simulink model "DAQ_v7_IMU_no_Boom_improved_differentiation"  (Simulink 7.8)
settings: Solver=ode3  StartTime=0.0  StopTime=inf  FixedStep=0.001  RelTol=1e-3
InitFcn:
  | DAQParams
model workspace: external: MATLAB File (data not in the file)
undefined symbols (not defined in the file or in its folder): A_dirty_deriv, A_dirty_deriv_IMU, B_dirty_deriv, B_dirty_deriv_IMU, C_dirty_deriv, C_dirty_deriv_IMU, CalParams, D_dirty_deriv, D_dirty_deriv_IMU, Dt_dirty_deriv, Dt_dirty_deriv_IMU, IMU_Alignment_Params, MotorParams, x0_dirty_deriv, x0_dirty_deriv_IMU
libraries: xpcethercatlib x169, dspswit3 x1
(part 1 of 3)
settings Model: xpc_rtwmakecfg_data=_xpcethercatlib_  Creator=hareen  LastModifiedBy=kevinsg  SimulationMode=external  BufferReuse=off
settings DataIOCC: MaxDataPoints=1000000000  SaveFormat=StructureWithTime  SaveState=on
settings OptimizationCC: BlockReduction=off  OptimizeBlockIOStorage=off  BufferReuse=off  ExpressionFolding=off  LocalBlockOutputs=off
settings DebuggingCC: FcnCallInpInsideContextMsg=Use local settings
settings HardwareCC: ProdIntDivRoundTo=Zero  ProdEndianess=LittleEndian  ProdHWDeviceType=Generic->32-bit x86 compatible
settings RTWCC: SystemTargetFile=xpctarget.tlc  TemplateMakefile=xpc_default_tmf  Description=xPC Target  RTWVerbose=off  ProcessScript=xpctarget_make_rtw_hook  RTWCompilerOptimization=On
settings xpcTargetCC: TargetFcnLib=ansi_tfl_table_tmw.mat  TargetFunctionLibrary=XPC_BLAS  CodeExecutionProfiling=off  ParMdlRefBuildCompliant=on  ConcurrentExecutionCompliant=on  CombineSignalStateStructs=off  PortableWordSizes=off  RL32LogBufSizeModifier=10000000  xPCTaskExecutionProfile=off  xPCRL32EventNumber=5000  xPCLoadParamSetFile=off  xPCConcurrentTasks=off  xPCEnableSFAnimation=off

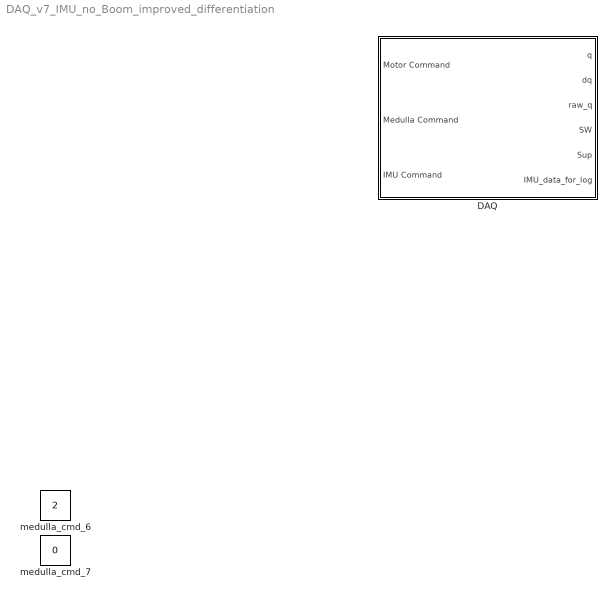
== system DAQ_v7_IMU_no_Boom_improved_differentiation ==
  DAQ : Subsystem
  medulla_cmd_6 : Constant  Value=2
  medulla_cmd_7 : Constant  Value=0

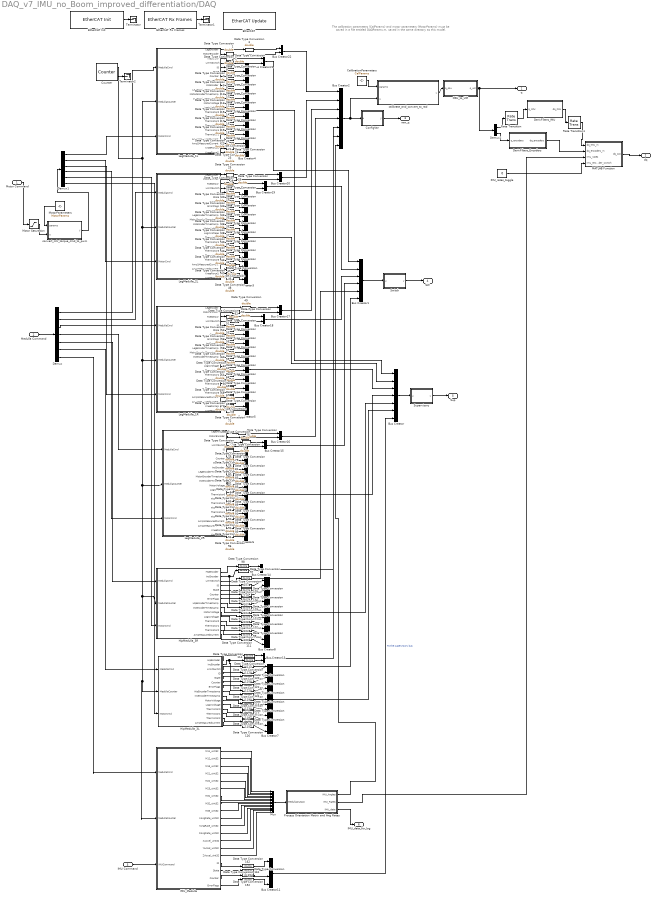
== system DAQ_v7_IMU_no_Boom_improved_differentiation/DAQ ==
  note: The calibration parameters (CalParams) and motor parameters (MotorParams)
      | must be saved in a file entitled DAQParams.m, saved in the same directory
      | as this model.
  Motor Command : Inport
  Medulla Command : Inport  Port=2
  IMU Command : Inport  Port=3
  Bus Creator : BusCreator  Inputs=7
  Bus Creator1 : BusCreator  Inputs=6
  Bus Creator11 : BusCreator
  Bus Creator{13..22} (10 alike) : BusCreator  Inputs=2
  Bus Creator2 : BusCreator  Inputs=7
  Bus Creator{3..6} (4 alike) : BusCreator  Inputs=20
  Bus Creator7 : BusCreator  Inputs=13
  Bus Creator8 : BusCreator  Inputs=13
  CalibrationParameters : Constant  Value=CalParams
  ConfigVar : MATLAB Function  TreatAsAtomicUnit=on
  Counter : dspswit3/Counter  Direction=Up  CountEvent=Free running  CounterSize=User defined  MaxCount=65535  InitialCount=0  Output=Count and Hit  HitValue=32  ResetInput=off  SamplesPerFrame=1  Ts=.001  CntDtype=double  HitDtype=Logical
  Data Type Conversion{1..126,152,154,157..158,161..162} (132 alike) : DataTypeConversion  OutDataTypeStr=double
  Demux : Demux  Outputs=7
  Demux1 : Demux  Outputs=6
  Demux2 : Demux  Outputs=[3 10]
  DerivFilters_Encoders : Subsystem
  DerivFilters_IMU : Subsystem
  EtherCAT : xpcethercatlib/EtherCAT Update   Priority=4  device_id=0  task_id_list=[1]  task_rates=[1]  task_priorities=[1500]  is_async=on  async_rates=20  async_priority=0
  EtherCAT Init : xpcethercatlib/EtherCAT Init   Priority=0  config_file='full_robot_eni_v5_no_boom.xml'  device_id=0  pci_bus=5  pci_slot=5  enaDC=on  errRptLevel=0  sample_time=-1
  EtherCAT Rx Frames : xpcethercatlib/EtherCAT Rx Frames   Priority=1  device_id=0  sample_time=0
  HipMedulla_3L : Subsystem
  HipMedulla_3R : Subsystem
  IMU_Medulla : Subsystem
  IMU_rates_toggle : Constant  Value=0
  LegMedulla_1L : Subsystem
  LegMedulla_1R : Subsystem
  LegMedulla_2L : Subsystem
  LegMedulla_2R : Subsystem
  MATLAB Function : MATLAB Function  TreatAsAtomicUnit=on
  Motor Saturation : Saturate  UpperLimit=50  LowerLimit=-50
  MotorParameters : Constant  Value=MotorParams
  Mux : Mux  Inputs=15
  OSU_to_UM : MATLAB Function  TreatAsAtomicUnit=on
  Process Orientation Matrix and Ang Rates : Subsystem
  Rate Transition : RateTransition  OutPortSampleTimeMultiple=2
  Rate Transition1 : RateTransition  Deterministic=off  OutPortSampleTime=.001
  Supervisory : MATLAB Function  TreatAsAtomicUnit=on
  Switch : MATLAB Function  TreatAsAtomicUnit=on
  Terminator : Terminator
  Terminator1 : Terminator
  Terminator2 : Terminator
  calibrate_and_convert_to_rad : MATLAB Function  TreatAsAtomicUnit=on
  convert_mtr_torque_cmd_to_pwm : MATLAB Function  TreatAsAtomicUnit=on
  q : Outport
  dq : Outport  Port=2
  raw_q : Outport  Port=3
  SW : Outport  Port=4
  Sup : Outport  Port=5
  IMU_data_for_log : Outport  Port=6
  wires:
  LegMedulla_1L/2(MotorEncoder) -> Data Type Conversion1/1
  LegMedulla_1L/3(ToeSensor) -> Data Type Conversion2/1
  LegMedulla_1L/4(LimitSwitch) -> Data Type Conversion4/1
  LegMedulla_1L/5(ID) -> Data Type Conversion5/1
  LegMedulla_1L/6(State) -> Data Type Conversion6/1
  LegMedulla_1L/7(Counter) -> Data Type Conversion7/1
  LegMedulla_1L/8(ErrorFlags) -> Data Type Conversion8/1
  LegMedulla_1L/9(IncEncoder) -> Data Type Conversion9/1
  LegMedulla_1L/10(LegEncoderTimestamp) -> Data Type Conversion10/1
  LegMedulla_1L/11(MotorEncoderTimestamp) -> Data Type Conversion11/1
  LegMedulla_1L/12(IncEncoderTimestamp) -> Data Type Conversion12/1
  LegMedulla_1L/13(MotorVoltage) -> Data Type Conversion13/1
  LegMedulla_1L/14(LogicVoltage) -> Data Type Conversion14/1
  LegMedulla_1L/15(Thermistor0) -> Data Type Conversion15/1
  LegMedulla_1L/16(Thermistor1) -> Data Type Conversion16/1
  LegMedulla_1L/17(Thermistor2) -> Data Type Conversion17/1
  LegMedulla_1L/18(Thermistor3) -> Data Type Conversion18/1
  LegMedulla_1L/19(Thermistor4) -> Data Type Conversion19/1
  LegMedulla_1L/20(Thermistor5) -> Data Type Conversion20/1
  LegMedulla_1L/21(Amp1MeasuredCurrent) -> Data Type Conversion21/1
  LegMedulla_1L/22(Amp2MeasuredCurrent) -> Data Type Conversion22/1
  LegMedulla_1L/23(KneeForce1) -> Data Type Conversion23/1
  LegMedulla_2L/1(LegEncoder) -> Data Type Conversion25/1
  LegMedulla_2L/2(MotorEncoder) -> Data Type Conversion26/1
  LegMedulla_2L/3(ToeSensor) -> Data Type Conversion27/1
  LegMedulla_2L/4(LimitSwitch) -> Data Type Conversion28/1
  LegMedulla_2L/5(ID) -> Data Type Conversion29/1
  LegMedulla_2L/6(State) -> Data Type Conversion30/1
  LegMedulla_2L/7(Counter) -> Data Type Conversion31/1
  LegMedulla_2L/8(ErrorFlags) -> Data Type Conversion32/1
  LegMedulla_2L/9(IncEncoder) -> Data Type Conversion33/1
  LegMedulla_2L/10(LegEncoderTimestamp) -> Data Type Conversion34/1
  LegMedulla_2L/11(MotorEncoderTimestamp) -> Data Type Conversion35/1
  LegMedulla_2L/12(IncEncoderTimestamp) -> Data Type Conversion36/1
  LegMedulla_2L/13(MotorVoltage) -> Data Type Conversion37/1
  LegMedulla_2L/14(LogicVoltage) -> Data Type Conversion38/1
  LegMedulla_2L/15(Thermistor0) -> Data Type Conversion39/1
  LegMedulla_2L/16(Thermistor1) -> Data Type Conversion40/1
  LegMedulla_2L/17(Thermistor2) -> Data Type Conversion41/1
  LegMedulla_2L/18(Thermistor3) -> Data Type Conversion42/1
  LegMedulla_2L/19(Thermistor4) -> Data Type Conversion43/1
  LegMedulla_2L/20(Thermistor5) -> Data Type Conversion44/1
  LegMedulla_2L/21(Amp1MeasuredCurrent) -> Data Type Conversion45/1
  LegMedulla_2L/22(Amp2MeasuredCurrent) -> Data Type Conversion46/1
  LegMedulla_2L/23(KneeForce1) -> Data Type Conversion47/1
  LegMedulla_1L/24(KneeForce2) -> Data Type Conversion24/1
  LegMedulla_2L/24(KneeForce2) -> Data Type Conversion48/1
  LegMedulla_1R/3(ToeSensor) -> Data Type Conversion51/1
  LegMedulla_1R/4(LimitSwitch) -> Data Type Conversion52/1
  LegMedulla_1R/5(ID) -> Data Type Conversion53/1
  LegMedulla_1R/6(State) -> Data Type Conversion54/1
  LegMedulla_1R/7(Counter) -> Data Type Conversion55/1
  LegMedulla_1R/8(ErrorFlags) -> Data Type Conversion56/1
  LegMedulla_1R/9(IncEncoder) -> Data Type Conversion57/1
  LegMedulla_1R/10(LegEncoderTimestamp) -> Data Type Conversion58/1
  LegMedulla_1R/11(MotorEncoderTimestamp) -> Data Type Conversion59/1
  LegMedulla_1R/12(IncEncoderTimestamp) -> Data Type Conversion60/1
  LegMedulla_1R/13(MotorVoltage) -> Data Type Conversion61/1
  LegMedulla_1R/14(LogicVoltage) -> Data Type Conversion62/1
  LegMedulla_1R/15(Thermistor0) -> Data Type Conversion63/1
  LegMedulla_1R/16(Thermistor1) -> Data Type Conversion64/1
  LegMedulla_1R/17(Thermistor2) -> Data Type Conversion65/1
  LegMedulla_1R/18(Thermistor3) -> Data Type Conversion66/1
  LegMedulla_1R/19(Thermistor4) -> Data Type Conversion67/1
  LegMedulla_1R/20(Thermistor5) -> Data Type Conversion68/1
  LegMedulla_1R/21(Amp1MeasuredCurrent) -> Data Type Conversion69/1
  LegMedulla_1R/22(Amp2MeasuredCurrent) -> Data Type Conversion70/1
  LegMedulla_1R/23(KneeForce1) -> Data Type Conversion71/1
  LegMedulla_2R/4(LimitSwitch) -> Data Type Conversion76/1
  LegMedulla_2R/5(ID) -> Data Type Conversion77/1
  LegMedulla_2R/6(State) -> Data Type Conversion78/1
  LegMedulla_2R/7(Counter) -> Data Type Conversion79/1
  LegMedulla_2R/8(ErrorFlags) -> Data Type Conversion80/1
  LegMedulla_2R/9(IncEncoder) -> Data Type Conversion81/1
  LegMedulla_2R/10(LegEncoderTimestamp) -> Data Type Conversion82/1
  LegMedulla_2R/11(MotorEncoderTimestamp) -> Data Type Conversion83/1
  LegMedulla_2R/12(IncEncoderTimestamp) -> Data Type Conversion84/1
  LegMedulla_2R/13(MotorVoltage) -> Data Type Conversion85/1
  LegMedulla_2R/14(LogicVoltage) -> Data Type Conversion86/1
  LegMedulla_2R/15(Thermistor0) -> Data Type Conversion87/1
  LegMedulla_2R/16(Thermistor1) -> Data Type Conversion88/1
  LegMedulla_2R/17(Thermistor2) -> Data Type Conversion89/1
  LegMedulla_2R/18(Thermistor3) -> Data Type Conversion90/1
  LegMedulla_2R/19(Thermistor4) -> Data Type Conversion91/1
  LegMedulla_2R/20(Thermistor5) -> Data Type Conversion92/1
  LegMedulla_2R/21(Amp1MeasuredCurrent) -> Data Type Conversion93/1
  LegMedulla_2R/22(Amp2MeasuredCurrent) -> Data Type Conversion94/1
  LegMedulla_2R/23(KneeForce1) -> Data Type Conversion95/1
  LegMedulla_1R/24(KneeForce2) -> Data Type Conversion72/1
  LegMedulla_2R/24(KneeForce2) -> Data Type Conversion96/1
  Counter/1 -> LegMedulla_1L/2(MedullaCounter), LegMedulla_2L/2(MedullaCounter), LegMedulla_1R/2(MedullaCounter), LegMedulla_2R/2(MedullaCounter), HipMedulla_3R/2(MedullaCounter), HipMedulla_3L/2(MedullaCounter), IMU_Medulla/2(MedullaCounter)
  Medulla Command/1 -> Demux/1
  Demux/1 -> LegMedulla_1L/1(MedullaCmd)
  Demux/2 -> LegMedulla_2L/1(MedullaCmd)
  Demux/3 -> LegMedulla_1R/1(MedullaCmd)
  Demux/4 -> LegMedulla_2R/1(MedullaCmd)
  Demux/5 -> HipMedulla_3R/1(MedullaCmd)
  Demux/6 -> HipMedulla_3L/1(MedullaCmd)
  Demux/7 -> IMU_Medulla/1(MedullaCmd)
  Demux1/1 -> LegMedulla_1L/3(MotorCmd)
  Demux1/2 -> LegMedulla_2L/3(MotorCmd)
  Demux1/3 -> LegMedulla_1R/3(MotorCmd)
  Demux1/4 -> LegMedulla_2R/3(MotorCmd)
  Demux1/5 -> HipMedulla_3R/3(MotorCmd)
  Demux1/6 -> HipMedulla_3L/3(MotorCmd)
  EtherCAT Init/1 -> Terminator/1
  EtherCAT Rx Frames/1 -> Terminator1/1
  Counter/2 -> Terminator2/1
  LegMedulla_2R/1(LegEncoder) -> Data Type Conversion73/1
  LegMedulla_2R/2(MotorEncoder) -> Data Type Conversion74/1
  LegMedulla_2R/3(ToeSensor) -> Data Type Conversion75/1
  Data Type Conversion51/1 -> Bus Creator18/1
  Data Type Conversion52/1 -> Bus Creator18/2
  Data Type Conversion53/1 -> Bus Creator5/1
  Data Type Conversion54/1 -> Bus Creator5/2
  Data Type Conversion55/1 -> Bus Creator5/3
  Data Type Conversion56/1 -> Bus Creator5/4
  Data Type Conversion57/1 -> Bus Creator5/5
  Data Type Conversion58/1 -> Bus Creator5/6
  Data Type Conversion59/1 -> Bus Creator5/7
  Data Type Conversion60/1 -> Bus Creator5/8
  Data Type Conversion61/1 -> Bus Creator5/9
  Data Type Conversion62/1 -> Bus Creator5/10
  Data Type Conversion63/1 -> Bus Creator5/11
  Data Type Conversion64/1 -> Bus Creator5/12
  Data Type Conversion65/1 -> Bus Creator5/13
  Data Type Conversion66/1 -> Bus Creator5/14
  Data Type Conversion67/1 -> Bus Creator5/15
  Data Type Conversion68/1 -> Bus Creator5/16
  Data Type Conversion69/1 -> Bus Creator5/17
  Data Type Conversion70/1 -> Bus Creator5/18
  Data Type Conversion71/1 -> Bus Creator5/19
  Data Type Conversion72/1 -> Bus Creator5/20
  Data Type Conversion73/1 -> Bus Creator16/1
  Data Type Conversion74/1 -> Bus Creator16/2
  Data Type Conversion75/1 -> Bus Creator15/1
  Data Type Conversion76/1 -> Bus Creator15/2
  Data Type Conversion77/1 -> Bus Creator6/1
  Data Type Conversion78/1 -> Bus Creator6/2
  Data Type Conversion79/1 -> Bus Creator6/3
  Data Type Conversion80/1 -> Bus Creator6/4
  Data Type Conversion81/1 -> Bus Creator6/5
  Data Type Conversion82/1 -> Bus Creator6/6
  Data Type Conversion83/1 -> Bus Creator6/7
  Data Type Conversion84/1 -> Bus Creator6/8
  Data Type Conversion85/1 -> Bus Creator6/9
  Data Type Conversion86/1 -> Bus Creator6/10
  Data Type Conversion87/1 -> Bus Creator6/11
  Data Type Conversion88/1 -> Bus Creator6/12
  Data Type Conversion89/1 -> Bus Creator6/13
  Data Type Conversion90/1 -> Bus Creator6/14
  Data Type Conversion91/1 -> Bus Creator6/15
  Data Type Conversion92/1 -> Bus Creator6/16
  Data Type Conversion93/1 -> Bus Creator6/17
  Data Type Conversion94/1 -> Bus Creator6/18
  Data Type Conversion95/1 -> Bus Creator6/19
  Data Type Conversion96/1 -> Bus Creator6/20
  Data Type Conversion111/1 -> Bus Creator8/13
  Motor Command/1 -> Motor Saturation/1
  MotorParameters/1 -> convert_mtr_torque_cmd_to_pwm/1(params)
  Motor Saturation/1 -> convert_mtr_torque_cmd_to_pwm/2(u)
  LegMedulla_1R/2(MotorEncoder) -> Data Type Conversion50/1
  LegMedulla_1L/1(LegEncoder) -> Data Type Conversion3/1
  LegMedulla_1R/1(LegEncoder) -> Data Type Conversion49/1
  Bus Creator22/1 -> Bus Creator2/1
  Bus Creator20/1 -> Bus Creator2/2
  Bus Creator17/1 -> Bus Creator2/3
  Bus Creator16/1 -> Bus Creator2/4
  Bus Creator14/1 -> Bus Creator2/5
  Bus Creator18/1 -> Bus Creator1/3
  Bus Creator19/1 -> Bus Creator1/2
  Bus Creator21/1 -> Bus Creator1/1
  Bus Creator15/1 -> Bus Creator1/4
  Data Type Conversion3/1 -> Bus Creator22/1
  Data Type Conversion1/1 -> Bus Creator22/2
  Data Type Conversion2/1 -> Bus Creator21/1
  Data Type Conversion4/1 -> Bus Creator21/2
  Data Type Conversion5/1 -> Bus Creator4/1
  Data Type Conversion6/1 -> Bus Creator4/2
  Data Type Conversion7/1 -> Bus Creator4/3
  Data Type Conversion8/1 -> Bus Creator4/4
  Data Type Conversion9/1 -> Bus Creator4/5
  Data Type Conversion10/1 -> Bus Creator4/6
  Data Type Conversion11/1 -> Bus Creator4/7
  Data Type Conversion12/1 -> Bus Creator4/8
  Data Type Conversion13/1 -> Bus Creator4/9
  Data Type Conversion14/1 -> Bus Creator4/10
  Data Type Conversion15/1 -> Bus Creator4/11
  Data Type Conversion16/1 -> Bus Creator4/12
  Data Type Conversion17/1 -> Bus Creator4/13
  Data Type Conversion18/1 -> Bus Creator4/14
  Data Type Conversion19/1 -> Bus Creator4/15
  Data Type Conversion20/1 -> Bus Creator4/16
  Data Type Conversion21/1 -> Bus Creator4/17
  Data Type Conversion22/1 -> Bus Creator4/18
  Data Type Conversion23/1 -> Bus Creator4/19
  Data Type Conversion24/1 -> Bus Creator4/20
  Data Type Conversion25/1 -> Bus Creator20/1
  Data Type Conversion26/1 -> Bus Creator20/2
  Data Type Conversion27/1 -> Bus Creator19/1
  Data Type Conversion28/1 -> Bus Creator19/2
  Data Type Conversion29/1 -> Bus Creator3/1
  Data Type Conversion30/1 -> Bus Creator3/2
  Data Type Conversion31/1 -> Bus Creator3/3
  Data Type Conversion32/1 -> Bus Creator3/4
  Data Type Conversion33/1 -> Bus Creator3/5
  Data Type Conversion34/1 -> Bus Creator3/6
  Data Type Conversion35/1 -> Bus Creator3/7
  Data Type Conversion36/1 -> Bus Creator3/8
  Data Type Conversion37/1 -> Bus Creator3/9
  Data Type Conversion38/1 -> Bus Creator3/10
  Data Type Conversion39/1 -> Bus Creator3/11
  Data Type Conversion40/1 -> Bus Creator3/12
  Data Type Conversion41/1 -> Bus Creator3/13
  Data Type Conversion42/1 -> Bus Creator3/14
  Data Type Conversion43/1 -> Bus Creator3/15
  Data Type Conversion44/1 -> Bus Creator3/16
  Data Type Conversion45/1 -> Bus Creator3/17
  Data Type Conversion46/1 -> Bus Creator3/18
  Data Type Conversion47/1 -> Bus Creator3/19
  Data Type Conversion48/1 -> Bus Creator3/20
  Data Type Conversion49/1 -> Bus Creator17/1
  Data Type Conversion50/1 -> Bus Creator17/2
  convert_mtr_torque_cmd_to_pwm/1(y) -> Demux1/1
  Data Type Conversion99/1 -> Bus Creator8/12
  Data Type Conversion100/1 -> Bus Creator8/11
  Data Type Conversion102/1 -> Bus Creator8/10
  Data Type Conversion103/1 -> Bus Creator8/9
  Data Type Conversion101/1 -> Bus Creator8/8
  Data Type Conversion108/1 -> Bus Creator8/7
  Data Type Conversion109/1 -> Bus Creator8/6
  Data Type Conversion104/1 -> Bus Creator8/5
  Data Type Conversion106/1 -> Bus Creator8/4
  Data Type Conversion107/1 -> Bus Creator8/3
  Data Type Conversion105/1 -> Bus Creator8/2
  Data Type Conversion110/1 -> Bus Creator8/1
  Data Type Conversion97/1 -> Bus Creator14/2
  Data Type Conversion98/1 -> Bus Creator14/1
  HipMedulla_3R/1(HipEncoder) -> Data Type Conversion98/1
  HipMedulla_3R/2(IncEncoder) -> Data Type Conversion97/1, Data Type Conversion104/1
  Data Type Conversion157/1 -> Bus Creator1/5
  HipMedulla_3R/3(LimitSwitch) -> Data Type Conversion157/1
  HipMedulla_3R/4(ID) -> Data Type Conversion110/1
  HipMedulla_3R/5(State) -> Data Type Conversion105/1
  HipMedulla_3R/6(Counter) -> Data Type Conversion107/1
  HipMedulla_3R/7(ErrorFlags) -> Data Type Conversion106/1
  HipMedulla_3R/8(HipEncoderTimestamp) -> Data Type Conversion109/1
  HipMedulla_3R/9(IncEncoderTimestamp) -> Data Type Conversion108/1
  HipMedulla_3R/10(MotorVoltage) -> Data Type Conversion101/1
  HipMedulla_3R/11(LogicVoltage) -> Data Type Conversion103/1
  HipMedulla_3R/12(Thermistor0) -> Data Type Conversion102/1
  HipMedulla_3R/13(Thermistor1) -> Data Type Conversion100/1
  HipMedulla_3R/14(Thermistor2) -> Data Type Conversion99/1
  HipMedulla_3R/15(AmpMeasuredCurrent) -> Data Type Conversion111/1
  Bus Creator13/1 -> Bus Creator2/6
  HipMedulla_3L/3(LimitSwitch) -> Data Type Conversion112/1
  Data Type Conversion112/1 -> Bus Creator1/6
  Data Type Conversion113/1 -> Bus Creator13/2
  Data Type Conversion114/1 -> Bus Creator13/1
  HipMedulla_3L/1(HipEncoder) -> Data Type Conversion114/1
  HipMedulla_3L/2(IncEncoder) -> Data Type Conversion113/1, Data Type Conversion119/1
  Data Type Conversion126/1 -> Bus Creator7/13
  Data Type Conversion158/1 -> Bus Creator7/12
  Data Type Conversion115/1 -> Bus Creator7/11
  Data Type Conversion117/1 -> Bus Creator7/10
  Data Type Conversion118/1 -> Bus Creator7/9
  Data Type Conversion116/1 -> Bus Creator7/8
  Data Type Conversion123/1 -> Bus Creator7/7
  Data Type Conversion124/1 -> Bus Creator7/6
  Data Type Conversion119/1 -> Bus Creator7/5
  Data Type Conversion121/1 -> Bus Creator7/4
  Data Type Conversion122/1 -> Bus Creator7/3
  Data Type Conversion120/1 -> Bus Creator7/2
  Data Type Conversion125/1 -> Bus Creator7/1
  HipMedulla_3L/4(ID) -> Data Type Conversion125/1
  HipMedulla_3L/5(State) -> Data Type Conversion120/1
  HipMedulla_3L/6(Counter) -> Data Type Conversion122/1
  HipMedulla_3L/7(ErrorFlags) -> Data Type Conversion121/1
  HipMedulla_3L/8(HipEncoderTimestamp) -> Data Type Conversion124/1
  HipMedulla_3L/9(IncEncoderTimestamp) -> Data Type Conversion123/1
  HipMedulla_3L/10(MotorVoltage) -> Data Type Conversion116/1
  HipMedulla_3L/11(LogicVoltage) -> Data Type Conversion118/1
  HipMedulla_3L/12(Thermistor0) -> Data Type Conversion117/1
  HipMedulla_3L/13(Thermistor1) -> Data Type Conversion115/1
  HipMedulla_3L/14(Thermistor2) -> Data Type Conversion158/1
  HipMedulla_3L/15(AmpMeasuredCurrent) -> Data Type Conversion126/1
  Bus Creator8/1 -> Bus Creator/5
  Bus Creator6/1 -> Bus Creator/4
  Bus Creator5/1 -> Bus Creator/3
  Bus Creator3/1 -> Bus Creator/2
  Bus Creator4/1 -> Bus Creator/1
  Bus Creator7/1 -> Bus Creator/6
  Bus Creator1/1 -> Switch/1(u)
  Bus Creator/1 -> Supervisory/1(u)
  Switch/1(y) -> SW/1
  Supervisory/1(y) -> Sup/1
  Bus Creator2/1 -> ConfigVar/1(u), calibrate_and_convert_to_rad/2(u)
  ConfigVar/1(y) -> raw_q/1
  CalibrationParameters/1 -> calibrate_and_convert_to_rad/1(params)
  calibrate_and_convert_to_rad/1(y) -> OSU_to_UM/1(q_osu)
  OSU_to_UM/1(q_um) -> q/1, Demux2/1
  Mux/1 -> Process Orientation Matrix and Ang Rates/1(MedullaOutput)
  Data Type Conversion154/1 -> Bus Creator11/4
  Data Type Conversion152/1 -> Bus Creator11/3
  Data Type Conversion161/1 -> Bus Creator11/2
  Data Type Conversion162/1 -> Bus Creator11/1
  Bus Creator11/1 -> Bus Creator/7  "To the supervisory bus"
  Process Orientation Matrix and Ang Rates/1(IMU_Angles) -> Bus Creator2/7
  Process Orientation Matrix and Ang Rates/3(IMU_data) -> IMU_data_for_log/1
  Process Orientation Matrix and Ang Rates/2(IMU_Rates) -> MATLAB Function/3(imu_rates)
  IMU_Medulla/1(M11_uint32) -> Mux/1
  IMU_Medulla/2(M12_uint32) -> Mux/2
  IMU_Medulla/3(M13_uint32) -> Mux/3
  IMU_Medulla/4(M21_uint32) -> Mux/4
  IMU_Medulla/5(M22_uint32) -> Mux/5
  IMU_Medulla/6(M23_uint32) -> Mux/6
  IMU_Medulla/7(M31_uint32) -> Mux/7
  IMU_Medulla/8(M32_uint32) -> Mux/8
  IMU_Medulla/9(M33_uint32) -> Mux/9
  IMU_Medulla/10(XAngRate_uint32) -> Mux/10
  IMU_Medulla/11(YAngRate_uint32) -> Mux/11
  IMU_Medulla/12(ZAngRate_uint32) -> Mux/12
  IMU_Medulla/13(XAccel_uint32) -> Mux/13
  IMU_Medulla/14(YAccel_uint32) -> Mux/14
  IMU_Medulla/15(ZAccel_uint32) -> Mux/15
  IMU_Medulla/19(ErrorFlags) -> Data Type Conversion154/1
  IMU_Medulla/18(Counter) -> Data Type Conversion152/1
  IMU_Medulla/17(State) -> Data Type Conversion161/1
  IMU_Medulla/16(ID) -> Data Type Conversion162/1
  IMU Command/1 -> IMU_Medulla/3(iMUCommand)
  MATLAB Function/1(dq_out) -> dq/1
  IMU_rates_toggle/1 -> MATLAB Function/4(imu_encoder_switch)
  Demux2/1 -> Rate Transition/1
  Demux2/2 -> DerivFilters_Encoders/1(q_encoders)
  DerivFilters_Encoders/1(dq_encoders) -> MATLAB Function/2(dq_encoders_in)
  Rate Transition/1 -> DerivFilters_IMU/1(q_IMU)
  DerivFilters_IMU/1(dq_IMU) -> Rate Transition1/1
  Rate Transition1/1 -> MATLAB Function/1(dq_IMU_in)

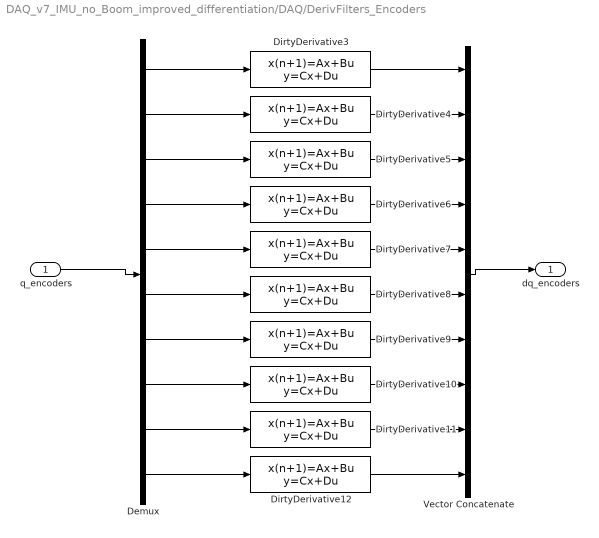
== system DAQ_v7_IMU_no_Boom_improved_differentiation/DAQ/DerivFilters_Encoders ==
  q_encoders : Inport
  Demux : Demux  Outputs=10
  DirtyDerivative{3..12} (10 alike) : DiscreteStateSpace  A=A_dirty_deriv  B=B_dirty_deriv  C=C_dirty_deriv  D=D_dirty_deriv  X0=x0_dirty_deriv  SampleTime=Dt_dirty_deriv
  Vector Concatenate : Concatenate  NumInputs=10  Mode=Vector
  dq_encoders : Outport
  wires:
  q_encoders/1 -> Demux/1
  Vector Concatenate/1 -> dq_encoders/1
  DirtyDerivative3/1 -> Vector Concatenate/1
  DirtyDerivative4/1 -> Vector Concatenate/2
  DirtyDerivative5/1 -> Vector Concatenate/3
  DirtyDerivative6/1 -> Vector Concatenate/4
  DirtyDerivative7/1 -> Vector Concatenate/5
  DirtyDerivative8/1 -> Vector Concatenate/6
  DirtyDerivative9/1 -> Vector Concatenate/7
  DirtyDerivative10/1 -> Vector Concatenate/8
  DirtyDerivative11/1 -> Vector Concatenate/9
  DirtyDerivative12/1 -> Vector Concatenate/10
  Demux/1 -> DirtyDerivative3/1
  Demux/2 -> DirtyDerivative4/1
  Demux/3 -> DirtyDerivative5/1
  Demux/4 -> DirtyDerivative6/1
  Demux/5 -> DirtyDerivative7/1
  Demux/6 -> DirtyDerivative8/1
  Demux/7 -> DirtyDerivative9/1
  Demux/8 -> DirtyDerivative10/1
  Demux/9 -> DirtyDerivative11/1
  Demux/10 -> DirtyDerivative12/1

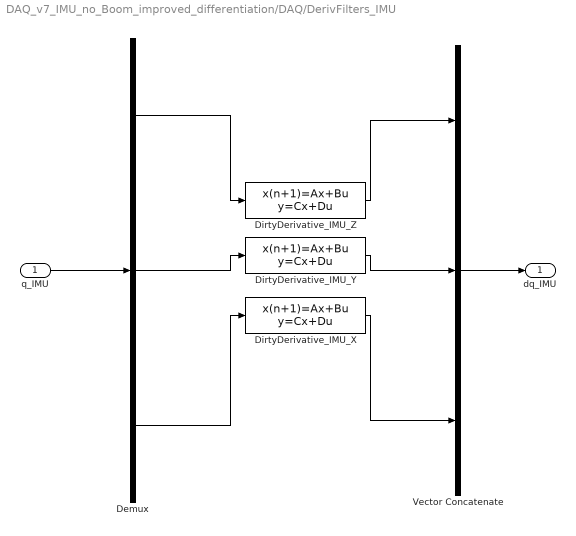
== system DAQ_v7_IMU_no_Boom_improved_differentiation/DAQ/DerivFilters_IMU ==
  q_IMU : Inport
  Demux : Demux  Outputs=3
  DirtyDerivative_IMU_X : DiscreteStateSpace  A=A_dirty_deriv_IMU  B=B_dirty_deriv_IMU  C=C_dirty_deriv_IMU  D=D_dirty_deriv_IMU  X0=x0_dirty_deriv_IMU  SampleTime=Dt_dirty_deriv_IMU
  DirtyDerivative_IMU_Y : DiscreteStateSpace  A=A_dirty_deriv_IMU  B=B_dirty_deriv_IMU  C=C_dirty_deriv_IMU  D=D_dirty_deriv_IMU  X0=x0_dirty_deriv_IMU  SampleTime=Dt_dirty_deriv_IMU
  DirtyDerivative_IMU_Z : DiscreteStateSpace  A=A_dirty_deriv_IMU  B=B_dirty_deriv_IMU  C=C_dirty_deriv_IMU  D=D_dirty_deriv_IMU  X0=x0_dirty_deriv_IMU  SampleTime=Dt_dirty_deriv_IMU
  Vector Concatenate : Concatenate  NumInputs=3  Mode=Vector
  dq_IMU : Outport
  wires:
  q_IMU/1 -> Demux/1
  Vector Concatenate/1 -> dq_IMU/1
  Demux/1 -> DirtyDerivative_IMU_Z/1
  DirtyDerivative_IMU_Z/1 -> Vector Concatenate/1
  DirtyDerivative_IMU_Y/1 -> Vector Concatenate/2
  DirtyDerivative_IMU_X/1 -> Vector Concatenate/3
  Demux/2 -> DirtyDerivative_IMU_Y/1
  Demux/3 -> DirtyDerivative_IMU_X/1

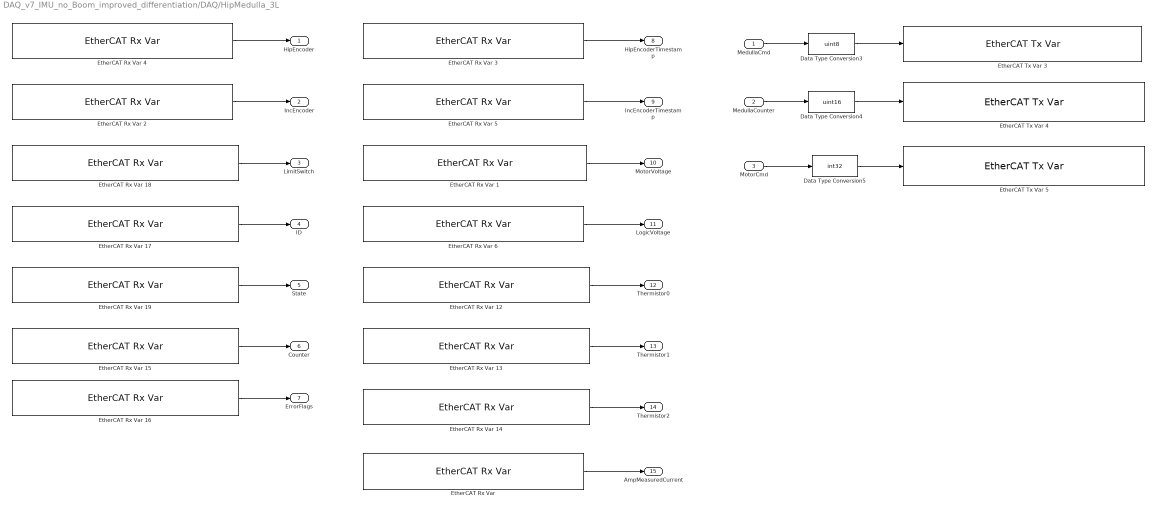
== system DAQ_v7_IMU_no_Boom_improved_differentiation/DAQ/HipMedulla_3L ==
  MedullaCmd : Inport
  MedullaCounter : Inport  Port=2
  MotorCmd : Inport  Port=3
  Data Type Conversion3 : DataTypeConversion  OutDataTypeStr=uint8
  Data Type Conversion4 : DataTypeConversion  OutDataTypeStr=uint16
  Data Type Conversion5 : DataTypeConversion  OutDataTypeStr=int32
  "EtherCAT Rx Var " : xpcethercatlib/EtherCAT Rx Var   Priority=2  sig_name=Box 6 (ATRIAS 2.1 Hip (Medulla 1.5)).Measured Current.Amp Measured Current  sig_offset=2352  sig_type=int16  type_size=16  sig_dim=1  device_id=0  sample_time=0.001000
  EtherCAT Rx Var 1 : xpcethercatlib/EtherCAT Rx Var   Priority=2  sig_name=Box 6 (ATRIAS 2.1 Hip (Medulla 1.5)).Power.Motor Voltage  sig_offset=2272  sig_type=uint16  type_size=16  sig_dim=1  device_id=0  sample_time=0.001000
  EtherCAT Rx Var 12 : xpcethercatlib/EtherCAT Rx Var   Priority=2  sig_name=Box 6 (ATRIAS 2.1 Hip (Medulla 1.5)).Thermistors.Thermistor 0  sig_offset=2304  sig_type=uint16  type_size=16  sig_dim=1  device_id=0  sample_time=0.001000
  EtherCAT Rx Var 13 : xpcethercatlib/EtherCAT Rx Var   Priority=2  sig_name=Box 6 (ATRIAS 2.1 Hip (Medulla 1.5)).Thermistors.Thermistor 1  sig_offset=2320  sig_type=uint16  type_size=16  sig_dim=1  device_id=0  sample_time=0.001000
  EtherCAT Rx Var 14 : xpcethercatlib/EtherCAT Rx Var   Priority=2  sig_name=Box 6 (ATRIAS 2.1 Hip (Medulla 1.5)).Thermistors.Thermistor 2  sig_offset=2336  sig_type=uint16  type_size=16  sig_dim=1  device_id=0  sample_time=0.001000
  EtherCAT Rx Var 15 : xpcethercatlib/EtherCAT Rx Var   Priority=2  sig_name=Box 6 (ATRIAS 2.1 Hip (Medulla 1.5)).uController Status.Counter  sig_offset=2200  sig_type=uint8  type_size=8  sig_dim=1  device_id=0  sample_time=0.001000
  EtherCAT Rx Var 16 : xpcethercatlib/EtherCAT Rx Var   Priority=2  sig_name=Box 6 (ATRIAS 2.1 Hip (Medulla 1.5)).uController Status.Error Flags  sig_offset=2208  sig_type=uint8  type_size=8  sig_dim=1  device_id=0  sample_time=0.001000
  EtherCAT Rx Var 17 : xpcethercatlib/EtherCAT Rx Var   Priority=2  sig_name=Box 6 (ATRIAS 2.1 Hip (Medulla 1.5)).uController Status.ID  sig_offset=2184  sig_type=uint8  type_size=8  sig_dim=1  device_id=0  sample_time=0.001000
  EtherCAT Rx Var 18 : xpcethercatlib/EtherCAT Rx Var   Priority=2  sig_name=Box 6 (ATRIAS 2.1 Hip (Medulla 1.5)).uController Status.Limit Switch  sig_offset=2216  sig_type=uint8  type_size=8  sig_dim=1  device_id=0  sample_time=0.001000
  EtherCAT Rx Var 19 : xpcethercatlib/EtherCAT Rx Var   Priority=2  sig_name=Box 6 (ATRIAS 2.1 Hip (Medulla 1.5)).uController Status.State  sig_offset=2192  sig_type=uint8  type_size=8  sig_dim=1  device_id=0  sample_time=0.001000
  EtherCAT Rx Var 2 : xpcethercatlib/EtherCAT Rx Var   Priority=2  sig_name=Box 6 (ATRIAS 2.1 Hip (Medulla 1.5)).Incremental Encoder.Incremental Encoder  sig_offset=2368  sig_type=uint16  type_size=16  sig_dim=1  device_id=0  sample_time=0.001000
  EtherCAT Rx Var 3 : xpcethercatlib/EtherCAT Rx Var   Priority=2  sig_name=Box 6 (ATRIAS 2.1 Hip (Medulla 1.5)).Hip Encoder.Timestamp  sig_offset=2256  sig_type=uint16  type_size=16  sig_dim=1  device_id=0  sample_time=0.001000
  EtherCAT Rx Var 4 : xpcethercatlib/EtherCAT Rx Var   Priority=2  sig_name=Box 6 (ATRIAS 2.1 Hip (Medulla 1.5)).Hip Encoder.Encoder  sig_offset=2224  sig_type=uint32  type_size=32  sig_dim=1  device_id=0  sample_time=0.001000
  EtherCAT Rx Var 5 : xpcethercatlib/EtherCAT Rx Var   Priority=2  sig_name=Box 6 (ATRIAS 2.1 Hip (Medulla 1.5)).Incremental Encoder.Incremental Encoder Timestamp  sig_offset=2384  sig_type=uint16  type_size=16  sig_dim=1  device_id=0  sample_time=0.001000
  EtherCAT Rx Var 6 : xpcethercatlib/EtherCAT Rx Var   Priority=2  sig_name=Box 6 (ATRIAS 2.1 Hip (Medulla 1.5)).Power.Logic Voltage  sig_offset=2288  sig_type=uint16  type_size=16  sig_dim=1  device_id=0  sample_time=0.001000
  EtherCAT Tx Var 3 : xpcethercatlib/EtherCAT Tx Var   Priority=3  sig_name=Box 6 (ATRIAS 2.1 Hip (Medulla 1.5)).uControllerInput.Command  sig_offset=2184  sig_type=uint8  type_size=8  sig_dim=1  device_id=0  sample_time=0.001000
  EtherCAT Tx Var 4 : xpcethercatlib/EtherCAT Tx Var   Priority=3  sig_name=Box 6 (ATRIAS 2.1 Hip (Medulla 1.5)).uControllerInput.Counter  sig_offset=2192  sig_type=uint16  type_size=16  sig_dim=1  device_id=0  sample_time=0.001000
  EtherCAT Tx Var 5 : xpcethercatlib/EtherCAT Tx Var   Priority=3  sig_name=Box 6 (ATRIAS 2.1 Hip (Medulla 1.5)).uControllerInput.Motor Current  sig_offset=2208  sig_type=int32  type_size=32  sig_dim=1  device_id=0  sample_time=0.001000
  HipEncoder : Outport
  IncEncoder : Outport  Port=2
  LimitSwitch : Outport  Port=3
  ID : Outport  Port=4
  State : Outport  Port=5
  Counter : Outport  Port=6
  ErrorFlags : Outport  Port=7
  HipEncoderTimestamp : Outport  Port=8
  IncEncoderTimestamp : Outport  Port=9
  MotorVoltage : Outport  Port=10
  LogicVoltage : Outport  Port=11
  Thermistor0 : Outport  Port=12
  Thermistor1 : Outport  Port=13
  Thermistor2 : Outport  Port=14
  AmpMeasuredCurrent : Outport  Port=15
  wires:
  Data Type Conversion3/1 -> EtherCAT Tx Var 3/1
  Data Type Conversion4/1 -> EtherCAT Tx Var 4/1
  Data Type Conversion5/1 -> EtherCAT Tx Var 5/1
  MedullaCmd/1 -> Data Type Conversion3/1
  MedullaCounter/1 -> Data Type Conversion4/1
  MotorCmd/1 -> Data Type Conversion5/1
  EtherCAT Rx Var 5/1 -> IncEncoderTimestamp/1
  EtherCAT Rx Var 4/1 -> HipEncoder/1
  EtherCAT Rx Var 3/1 -> HipEncoderTimestamp/1
  EtherCAT Rx Var 2/1 -> IncEncoder/1
  EtherCAT Rx Var 15/1 -> Counter/1
  EtherCAT Rx Var 17/1 -> ID/1
  EtherCAT Rx Var 18/1 -> LimitSwitch/1
  EtherCAT Rx Var 19/1 -> State/1
  EtherCAT Rx Var 16/1 -> ErrorFlags/1
  EtherCAT Rx Var 6/1 -> LogicVoltage/1
  EtherCAT Rx Var 1/1 -> MotorVoltage/1
  EtherCAT Rx Var 12/1 -> Thermistor0/1
  EtherCAT Rx Var 13/1 -> Thermistor1/1
  EtherCAT Rx Var 14/1 -> Thermistor2/1
  "EtherCAT Rx Var "/1 -> AmpMeasuredCurrent/1

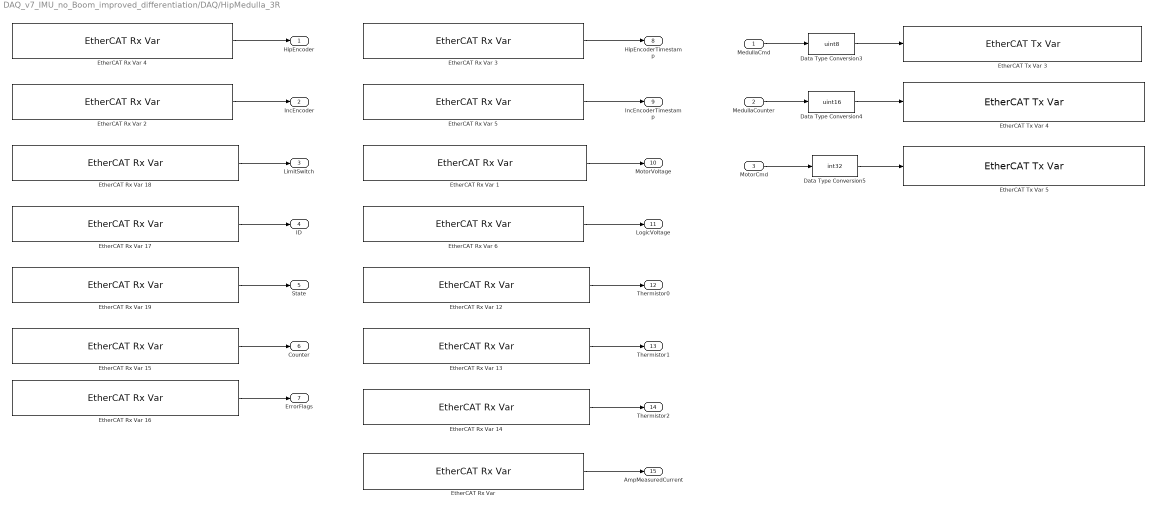
== system DAQ_v7_IMU_no_Boom_improved_differentiation/DAQ/HipMedulla_3R ==
  MedullaCmd : Inport
  MedullaCounter : Inport  Port=2
  MotorCmd : Inport  Port=3
  Data Type Conversion3 : DataTypeConversion  OutDataTypeStr=uint8
  Data Type Conversion4 : DataTypeConversion  OutDataTypeStr=uint16
  Data Type Conversion5 : DataTypeConversion  OutDataTypeStr=int32
  "EtherCAT Rx Var " : xpcethercatlib/EtherCAT Rx Var   Priority=2  sig_name=Box 5 (ATRIAS 2.1 Hip (Medulla 1.5)).Measured Current.Amp Measured Current  sig_offset=2136  sig_type=int16  type_size=16  sig_dim=1  device_id=0  sample_time=0.001000
  EtherCAT Rx Var 1 : xpcethercatlib/EtherCAT Rx Var   Priority=2  sig_name=Box 5 (ATRIAS 2.1 Hip (Medulla 1.5)).Power.Motor Voltage  sig_offset=2056  sig_type=uint16  type_size=16  sig_dim=1  device_id=0  sample_time=0.001000
  EtherCAT Rx Var 12 : xpcethercatlib/EtherCAT Rx Var   Priority=2  sig_name=Box 5 (ATRIAS 2.1 Hip (Medulla 1.5)).Thermistors.Thermistor 0  sig_offset=2088  sig_type=uint16  type_size=16  sig_dim=1  device_id=0  sample_time=0.001000
  EtherCAT Rx Var 13 : xpcethercatlib/EtherCAT Rx Var   Priority=2  sig_name=Box 5 (ATRIAS 2.1 Hip (Medulla 1.5)).Thermistors.Thermistor 1  sig_offset=2104  sig_type=uint16  type_size=16  sig_dim=1  device_id=0  sample_time=0.001000
  EtherCAT Rx Var 14 : xpcethercatlib/EtherCAT Rx Var   Priority=2  sig_name=Box 5 (ATRIAS 2.1 Hip (Medulla 1.5)).Thermistors.Thermistor 2  sig_offset=2120  sig_type=uint16  type_size=16  sig_dim=1  device_id=0  sample_time=0.001000
  EtherCAT Rx Var 15 : xpcethercatlib/EtherCAT Rx Var   Priority=2  sig_name=Box 5 (ATRIAS 2.1 Hip (Medulla 1.5)).uController Status.Counter  sig_offset=1984  sig_type=uint8  type_size=8  sig_dim=1  device_id=0  sample_time=0.001000
  EtherCAT Rx Var 16 : xpcethercatlib/EtherCAT Rx Var   Priority=2  sig_name=Box 5 (ATRIAS 2.1 Hip (Medulla 1.5)).uController Status.Error Flags  sig_offset=1992  sig_type=uint8  type_size=8  sig_dim=1  device_id=0  sample_time=0.001000
  EtherCAT Rx Var 17 : xpcethercatlib/EtherCAT Rx Var   Priority=2  sig_name=Box 5 (ATRIAS 2.1 Hip (Medulla 1.5)).uController Status.ID  sig_offset=1968  sig_type=uint8  type_size=8  sig_dim=1  device_id=0  sample_time=0.001000
  EtherCAT Rx Var 18 : xpcethercatlib/EtherCAT Rx Var   Priority=2  sig_name=Box 5 (ATRIAS 2.1 Hip (Medulla 1.5)).uController Status.Limit Switch  sig_offset=2000  sig_type=uint8  type_size=8  sig_dim=1  device_id=0  sample_time=0.001000
  EtherCAT Rx Var 19 : xpcethercatlib/EtherCAT Rx Var   Priority=2  sig_name=Box 5 (ATRIAS 2.1 Hip (Medulla 1.5)).uController Status.State  sig_offset=1976  sig_type=uint8  type_size=8  sig_dim=1  device_id=0  sample_time=0.001000
  EtherCAT Rx Var 2 : xpcethercatlib/EtherCAT Rx Var   Priority=2  sig_name=Box 5 (ATRIAS 2.1 Hip (Medulla 1.5)).Incremental Encoder.Incremental Encoder  sig_offset=2152  sig_type=uint16  type_size=16  sig_dim=1  device_id=0  sample_time=0.001000
  EtherCAT Rx Var 3 : xpcethercatlib/EtherCAT Rx Var   Priority=2  sig_name=Box 5 (ATRIAS 2.1 Hip (Medulla 1.5)).Hip Encoder.Timestamp  sig_offset=2040  sig_type=uint16  type_size=16  sig_dim=1  device_id=0  sample_time=0.001000
  EtherCAT Rx Var 4 : xpcethercatlib/EtherCAT Rx Var   Priority=2  sig_name=Box 5 (ATRIAS 2.1 Hip (Medulla 1.5)).Hip Encoder.Encoder  sig_offset=2008  sig_type=uint32  type_size=32  sig_dim=1  device_id=0  sample_time=0.001000
  EtherCAT Rx Var 5 : xpcethercatlib/EtherCAT Rx Var   Priority=2  sig_name=Box 5 (ATRIAS 2.1 Hip (Medulla 1.5)).Incremental Encoder.Incremental Encoder Timestamp  sig_offset=2168  sig_type=uint16  type_size=16  sig_dim=1  device_id=0  sample_time=0.001000
  EtherCAT Rx Var 6 : xpcethercatlib/EtherCAT Rx Var   Priority=2  sig_name=Box 5 (ATRIAS 2.1 Hip (Medulla 1.5)).Power.Logic Voltage  sig_offset=2072  sig_type=uint16  type_size=16  sig_dim=1  device_id=0  sample_time=0.001000
  EtherCAT Tx Var 3 : xpcethercatlib/EtherCAT Tx Var   Priority=3  sig_name=Box 5 (ATRIAS 2.1 Hip (Medulla 1.5)).uControllerInput.Command  sig_offset=1968  sig_type=uint8  type_size=8  sig_dim=1  device_id=0  sample_time=0.001000
  EtherCAT Tx Var 4 : xpcethercatlib/EtherCAT Tx Var   Priority=3  sig_name=Box 5 (ATRIAS 2.1 Hip (Medulla 1.5)).uControllerInput.Counter  sig_offset=1976  sig_type=uint16  type_size=16  sig_dim=1  device_id=0  sample_time=0.001000
  EtherCAT Tx Var 5 : xpcethercatlib/EtherCAT Tx Var   Priority=3  sig_name=Box 5 (ATRIAS 2.1 Hip (Medulla 1.5)).uControllerInput.Motor Current  sig_offset=1992  sig_type=int32  type_size=32  sig_dim=1  device_id=0  sample_time=0.001000
  HipEncoder : Outport
  IncEncoder : Outport  Port=2
  LimitSwitch : Outport  Port=3
  ID : Outport  Port=4
  State : Outport  Port=5
  Counter : Outport  Port=6
  ErrorFlags : Outport  Port=7
  HipEncoderTimestamp : Outport  Port=8
  IncEncoderTimestamp : Outport  Port=9
  MotorVoltage : Outport  Port=10
  LogicVoltage : Outport  Port=11
  Thermistor0 : Outport  Port=12
  Thermistor1 : Outport  Port=13
  Thermistor2 : Outport  Port=14
  AmpMeasuredCurrent : Outport  Port=15
  wires:
  Data Type Conversion3/1 -> EtherCAT Tx Var 3/1
  Data Type Conversion4/1 -> EtherCAT Tx Var 4/1
  Data Type Conversion5/1 -> EtherCAT Tx Var 5/1
  MedullaCmd/1 -> Data Type Conversion3/1
  MedullaCounter/1 -> Data Type Conversion4/1
  MotorCmd/1 -> Data Type Conversion5/1
  EtherCAT Rx Var 5/1 -> IncEncoderTimestamp/1
  EtherCAT Rx Var 4/1 -> HipEncoder/1
  EtherCAT Rx Var 3/1 -> HipEncoderTimestamp/1
  EtherCAT Rx Var 2/1 -> IncEncoder/1
  EtherCAT Rx Var 15/1 -> Counter/1
  EtherCAT Rx Var 17/1 -> ID/1
  EtherCAT Rx Var 18/1 -> LimitSwitch/1
  EtherCAT Rx Var 19/1 -> State/1
  EtherCAT Rx Var 16/1 -> ErrorFlags/1
  EtherCAT Rx Var 6/1 -> LogicVoltage/1
  EtherCAT Rx Var 1/1 -> MotorVoltage/1
  EtherCAT Rx Var 12/1 -> Thermistor0/1
  EtherCAT Rx Var 13/1 -> Thermistor1/1
  EtherCAT Rx Var 14/1 -> Thermistor2/1
  "EtherCAT Rx Var "/1 -> AmpMeasuredCurrent/1

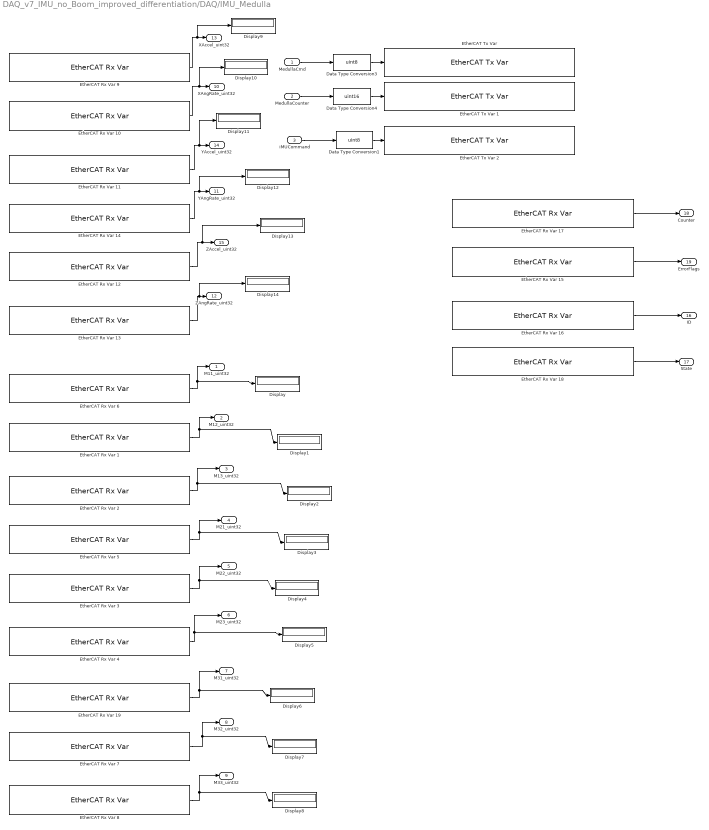
== system DAQ_v7_IMU_no_Boom_improved_differentiation/DAQ/IMU_Medulla ==
  MedullaCmd : Inport
  MedullaCounter : Inport  Port=2
  iMUCommand : Inport  Port=3
  Data Type Conversion1 : DataTypeConversion  OutDataTypeStr=uint8
  Data Type Conversion3 : DataTypeConversion  OutDataTypeStr=uint8
  Data Type Conversion4 : DataTypeConversion  OutDataTypeStr=uint16
  Display{,1..14} (15 alike) : Display
  EtherCAT Rx Var 1 : xpcethercatlib/EtherCAT Rx Var   Priority=2  sig_name=Box 8 (ATRIAS 2.1 Leg (Medulla 1.5)).M.M12  sig_offset=2656  sig_type=uint32  type_size=32  sig_dim=1  device_id=0  sample_time=0.001000
  EtherCAT Rx Var 10 : xpcethercatlib/EtherCAT Rx Var   Priority=2  sig_name=Box 8 (ATRIAS 2.1 Leg (Medulla 1.5)).Xaxes.XAngRate  sig_offset=2432  sig_type=uint32  type_size=32  sig_dim=1  device_id=0  sample_time=0.001000
  EtherCAT Rx Var 11 : xpcethercatlib/EtherCAT Rx Var   Priority=2  sig_name=Box 8 (ATRIAS 2.1 Leg (Medulla 1.5)).Yaxes.YAccel  sig_offset=2528  sig_type=uint32  type_size=32  sig_dim=1  device_id=0  sample_time=0.001000
  EtherCAT Rx Var 12 : xpcethercatlib/EtherCAT Rx Var   Priority=2  sig_name=Box 8 (ATRIAS 2.1 Leg (Medulla 1.5)).Zaxes.ZAccel  sig_offset=2592  sig_type=uint32  type_size=32  sig_dim=1  device_id=0  sample_time=0.001000
  EtherCAT Rx Var 13 : xpcethercatlib/EtherCAT Rx Var   Priority=2  sig_name=Box 8 (ATRIAS 2.1 Leg (Medulla 1.5)).Zaxes.ZAngRate  sig_offset=2560  sig_type=uint32  type_size=32  sig_dim=1  device_id=0  sample_time=0.001000
  EtherCAT Rx Var 14 : xpcethercatlib/EtherCAT Rx Var   Priority=2  sig_name=Box 8 (ATRIAS 2.1 Leg (Medulla 1.5)).Yaxes.YAngRate  sig_offset=2496  sig_type=uint32  type_size=32  sig_dim=1  device_id=0  sample_time=0.001000
  EtherCAT Rx Var 15 : xpcethercatlib/EtherCAT Rx Var   Priority=2  sig_name=Box 8 (ATRIAS 2.1 Leg (Medulla 1.5)).uController Status.Error Flags  sig_offset=2424  sig_type=uint8  type_size=8  sig_dim=1  device_id=0  sample_time=0.001000
  EtherCAT Rx Var 16 : xpcethercatlib/EtherCAT Rx Var   Priority=2  sig_name=Box 8 (ATRIAS 2.1 Leg (Medulla 1.5)).uController Status.ID  sig_offset=2400  sig_type=uint8  type_size=8  sig_dim=1  device_id=0  sample_time=0.001000
  EtherCAT Rx Var 17 : xpcethercatlib/EtherCAT Rx Var   Priority=2  sig_name=Box 8 (ATRIAS 2.1 Leg (Medulla 1.5)).uController Status.Counter  sig_offset=2416  sig_type=uint8  type_size=8  sig_dim=1  device_id=0  sample_time=0.001000
  EtherCAT Rx Var 18 : xpcethercatlib/EtherCAT Rx Var   Priority=2  sig_name=Box 8 (ATRIAS 2.1 Leg (Medulla 1.5)).uController Status.State  sig_offset=2408  sig_type=uint8  type_size=8  sig_dim=1  device_id=0  sample_time=0.001000
  EtherCAT Rx Var 19 : xpcethercatlib/EtherCAT Rx Var   Priority=2  sig_name=Box 8 (ATRIAS 2.1 Leg (Medulla 1.5)).M.M31  sig_offset=2816  sig_type=uint32  type_size=32  sig_dim=1  device_id=0  sample_time=0.001000
  EtherCAT Rx Var 2 : xpcethercatlib/EtherCAT Rx Var   Priority=2  sig_name=Box 8 (ATRIAS 2.1 Leg (Medulla 1.5)).M.M13  sig_offset=2688  sig_type=uint32  type_size=32  sig_dim=1  device_id=0  sample_time=0.001000
  EtherCAT Rx Var 3 : xpcethercatlib/EtherCAT Rx Var   Priority=2  sig_name=Box 8 (ATRIAS 2.1 Leg (Medulla 1.5)).M.M22  sig_offset=2752  sig_type=uint32  type_size=32  sig_dim=1  device_id=0  sample_time=0.001000
  EtherCAT Rx Var 4 : xpcethercatlib/EtherCAT Rx Var   Priority=2  sig_name=Box 8 (ATRIAS 2.1 Leg (Medulla 1.5)).M.M23  sig_offset=2784  sig_type=uint32  type_size=32  sig_dim=1  device_id=0  sample_time=0.001000
  EtherCAT Rx Var 5 : xpcethercatlib/EtherCAT Rx Var   Priority=2  sig_name=Box 8 (ATRIAS 2.1 Leg (Medulla 1.5)).M.M21  sig_offset=2720  sig_type=uint32  type_size=32  sig_dim=1  device_id=0  sample_time=0.001000
  EtherCAT Rx Var 6 : xpcethercatlib/EtherCAT Rx Var   Priority=2  sig_name=Box 8 (ATRIAS 2.1 Leg (Medulla 1.5)).M.M11  sig_offset=2624  sig_type=uint32  type_size=32  sig_dim=1  device_id=0  sample_time=0.001000
  EtherCAT Rx Var 7 : xpcethercatlib/EtherCAT Rx Var   Priority=2  sig_name=Box 8 (ATRIAS 2.1 Leg (Medulla 1.5)).M.M32  sig_offset=2848  sig_type=uint32  type_size=32  sig_dim=1  device_id=0  sample_time=0.001000
  EtherCAT Rx Var 8 : xpcethercatlib/EtherCAT Rx Var   Priority=2  sig_name=Box 8 (ATRIAS 2.1 Leg (Medulla 1.5)).M.M33  sig_offset=2880  sig_type=uint32  type_size=32  sig_dim=1  device_id=0  sample_time=0.001000
  EtherCAT Rx Var 9 : xpcethercatlib/EtherCAT Rx Var   Priority=2  sig_name=Box 8 (ATRIAS 2.1 Leg (Medulla 1.5)).Xaxes.XAccel  sig_offset=2464  sig_type=uint32  type_size=32  sig_dim=1  device_id=0  sample_time=0.001000
  "EtherCAT Tx Var " : xpcethercatlib/EtherCAT Tx Var   Priority=3  sig_name=Box 1 (ATRIAS 2.1 Leg (Medulla 1.5)).uControllerInput.Command  sig_offset=464  sig_type=uint8  type_size=8  sig_dim=1  device_id=0  sample_time=0.001000
  EtherCAT Tx Var 1 : xpcethercatlib/EtherCAT Tx Var   Priority=3  sig_name=Box 1 (ATRIAS 2.1 Leg (Medulla 1.5)).uControllerInput.Counter  sig_offset=472  sig_type=uint16  type_size=16  sig_dim=1  device_id=0  sample_time=0.001000
  EtherCAT Tx Var 2 : xpcethercatlib/EtherCAT Tx Var   Priority=3  sig_name=Box 1 (ATRIAS 2.1 Leg (Medulla 1.5)).uControllerInput.Command  sig_offset=464  sig_type=uint8  type_size=8  sig_dim=1  device_id=0  sample_time=0.001000
  M11_uint32 : Outport
  M12_uint32 : Outport  Port=2
  M13_uint32 : Outport  Port=3
  M21_uint32 : Outport  Port=4
  M22_uint32 : Outport  Port=5
  M23_uint32 : Outport  Port=6
  M31_uint32 : Outport  Port=7
  M32_uint32 : Outport  Port=8
  M33_uint32 : Outport  Port=9
  XAngRate_uint32 : Outport  Port=10
  YAngRate_uint32 : Outport  Port=11
  ZAngRate_uint32 : Outport  Port=12
  XAccel_uint32 : Outport  Port=13
  YAccel_uint32 : Outport  Port=14
  ZAccel_uint32 : Outport  Port=15
  ID : Outport  Port=16
  State : Outport  Port=17
  Counter : Outport  Port=18
  ErrorFlags : Outport  Port=19
  wires:
  EtherCAT Rx Var 9/1 -> XAccel_uint32/1, Display9/1
  EtherCAT Rx Var 10/1 -> XAngRate_uint32/1, Display10/1
  EtherCAT Rx Var 11/1 -> YAccel_uint32/1, Display11/1
  EtherCAT Rx Var 14/1 -> YAngRate_uint32/1, Display12/1
  EtherCAT Rx Var 12/1 -> ZAccel_uint32/1, Display13/1
  EtherCAT Rx Var 13/1 -> ZAngRate_uint32/1, Display14/1
  EtherCAT Rx Var 6/1 -> M11_uint32/1, Display/1
  EtherCAT Rx Var 1/1 -> M12_uint32/1, Display1/1
  EtherCAT Rx Var 2/1 -> M13_uint32/1, Display2/1
  EtherCAT Rx Var 5/1 -> M21_uint32/1, Display3/1
  EtherCAT Rx Var 3/1 -> M22_uint32/1, Display4/1
  EtherCAT Rx Var 4/1 -> M23_uint32/1, Display5/1
  EtherCAT Rx Var 19/1 -> M31_uint32/1, Display6/1
  EtherCAT Rx Var 7/1 -> M32_uint32/1, Display7/1
  EtherCAT Rx Var 8/1 -> M33_uint32/1, Display8/1
  Data Type Conversion3/1 -> "EtherCAT Tx Var "/1
  Data Type Conversion4/1 -> EtherCAT Tx Var 1/1
  MedullaCmd/1 -> Data Type Conversion3/1
  MedullaCounter/1 -> Data Type Conversion4/1
  iMUCommand/1 -> Data Type Conversion1/1
  Data Type Conversion1/1 -> EtherCAT Tx Var 2/1
  EtherCAT Rx Var 17/1 -> Counter/1
  EtherCAT Rx Var 15/1 -> ErrorFlags/1
  EtherCAT Rx Var 16/1 -> ID/1
  EtherCAT Rx Var 18/1 -> State/1
